simulink model "MenakaModel"  (R2022a)
settings: Solver=ode23tb  StartTime=0.0  StopTime=4  MaxStep=10/(60*24)  RelTol=1e-3
model workspace (MAT data in the model file):
  clima__A_c = 3295.16408265
  clima__A_f = 3100.53942116
  clima__G0 = [0.05; 0.00070738]
  clima__H = 7.9995824611
  clima__T0 = [287.15; 287.15; 287.15; 287.15]
  clima__T_ss = 280.150340169
  clima__alpha_c = 0.0100640347387
  clima__alpha_f = 0.0111385012129
  clima__alpha_i = 0.1
  clima__c_s = [1081 1081]
  clima__cd_c = 8736
  clima__d_c = 1.5
  clima__hour0 = 1
  clima__int_air_speed = 0.5
  clima__l_s = [0.1 0.1]
  clima__lam_s = [2.5 0.85]
  clima__minWindows = 0.299965865643
  clima__rhod_s = [2600 2500]
  clima__tau_c = 1
  crop__A_v = 2080
  crop__C = [0.01 0.001 0.01 0.01]
  crop__C_buf_max = 0.02
  crop__C_wv = 0.2
  crop__Chi_nutrients = [0.015625; 0.0104166666667; 0.00520833333333; 0.00208333333333; 0.00208333333333; 0.00104166666667; 0; 0]
  crop__N = [0; 0; 0; 0; 0; 0; 0; 0]
  crop__R = [0 0 0]
  crop__T_max_v = 40
  crop__T_max_v24 = 27
  crop__T_min_v = 6
  crop__T_min_v24 = 14
  crop__T_sum_end = 1035
  crop__T_v_start_fruit = 1100
  crop__Tsum = 0
  crop__Tv = 288
  crop__b_N_uptake = 0.5
  crop__c_fruit_g = 0.27
  crop__c_fruit_m = 2.3e-07
  crop__c_leaf_g = 0.28
  crop__c_leaf_m = 3.47e-07
  crop__c_stem_g = 0.3
  crop__c_stem_m = 1.47e-07
  crop__fraction_DM = 0.08
  crop__int_air_speed = 0.5
  crop__min_water_capacity = 0.1
  crop__plants_density = 2.1562
  crop__rg_fruit = 2e-07
  crop__rg_leaf = 9.5e-08
  crop__rg_stem = 7.4e-08
  crop__s_buforg_buf = -5000
  crop__s_max_T = 0.5793
  crop__s_max_T24 = 1.3904
  crop__s_min_T = -0.869
  crop__s_min_T24 = -1.1587
  heater__A_e = 0.0001
  heater__A_i = 0.008
  heater__T = 288
  heater__c = 5e-10
  heater__power = 60000000
  screen__Power = 100
  screen__Radthreshold = 900
  screen__beta = 2.23564167038e-14
  screen__gamma_max = 2.26308905438e-14
  screen__velocity = 0.333333333333
  subtrate__C_ws = 0.1
  subtrate__N = [0; 0; 0; 0; 0; 0; 0; 0]
  subtrate__Nmin_subs = 1e-09
  subtrate__Vmax_subs = 10
  subtrate__Vmin_subs = 0.01
  subtrate__sigma_max = 1
  subtrate__sigma_min = 1
  tomato__Cfruit0 = 0.001
  windows__AR = 19.9974923936
  windows__Power = 100
  windows__RadThreshold = 10
  windows__max_night = 10
  windows__tau = 600
undefined symbols (not defined in the file or in its folder): CO2_ppm_ext, Gain_control_Tv_mean, Gain_control_Tv_mean_superior, gain_max_night, GAIN_WIN, Hmax, Hstart, max_night, maxvelocity, RadTh_windows, Radthhold, shift_temp_heat, tau_win, tend_crop1, tend_crop2, tinit_crop1, tinit_crop2, Tmax, Tmax_mean, Tstart, Tven_max, Tven_start, WinAR
libraries: HORTISIM x26, simulink x6
(part 5 of 5)

== matlab function MenakaModel/Control System/PID - constant setpoints - Ti measure/Subsystem1/Triggered Subsystem/MATLAB Function ==
  data: T_min output; T_opt_min output; Tsum input; Rad input; THRad input; T_opt_max output; Tmax output
function [T_min,T_opt_min,T_opt_max,Tmax] = fcn(Tsum, Rad,THRad)


r = OptimalGrowthTemperature(Tsum,Rad,THRad);
r = r + 273.15;

T_min = r(1);
T_opt_min = r(2);
T_opt_max = r(3);
Tmax = r(4);


end
%

function x = OptimalGrowthTemperature(Tsum,Rad,THRad)
    if size(Tsum,2)~=1
       error('Tsum debe ser una columna') 
    end
    x = (Rad> THRad).*OptimalGrowthTemperatureDay(Tsum) + ...
        (Rad<= THRad).*OptimalGrowthTemperatureNight(Tsum);
end


function x = OptimalGrowthTemperatureDay(Tsum)
    if size(Tsum,2)~=1
       error('Tsum debe ser una columna') 
    end
    
%         % Tmin Topt_min Topt_max Tmax
%     x =   [11      18      25     40  ].*theta(400,Tsum) + ...
%           [12      21      24     35  ].*theta(Tsum,400).*theta(1800,Tsum) + ...
%           [15      20      25     30  ].*theta(Tsum,1800);  
%       
              % Tmin Topt_min Topt_max Tmax
    x =   [11      18      35     40  ].*theta(400,Tsum) + ...
          [12      21      30     35  ].*theta(Tsum,400).*theta(1800,Tsum) + ...
          [15      20      30     30  ].*theta(Tsum,1800); 
end

function x = OptimalGrowthTemperatureNight(Tsum)
    if size(Tsum,2)~=1
       error('Tsum debe ser una columna') 
    end
%     x = [11 15 18 30 ].*theta(400,Tsum) + ...
%         [13 14 14 14].*theta(Tsum,400).*theta(1800,Tsum) + ...
%         [10 14 30 35].*theta(Tsum,1800);  
    
        x = [11 15 18 30 ].*theta(400,Tsum) + ...
            [12 13 15 16 ].*theta(Tsum,400).*theta(1800,Tsum) + ...
            [10 14 30 35 ].*theta(Tsum,1800);  
end


function r = theta(x,y)
    eta = 10;
    r = 0.5 + 0.5*tanh(eta*(x-y));
end

== matlab function MenakaModel/Control System/PID - constant setpoints - Ti measure/Subsystem1/Windows Controler/Subsystem/Selection  ==
  data: Rad input; Temperature input; y output; Humidity input; Rad_threshold input
function y = fcn(Rad,Temperature,Humidity,Rad_threshold)

h = double(Rad > Rad_threshold);

y = h*Temperature + (1-h)*Humidity;

%y = Temperature;

== matlab function MenakaModel/Control System/PID-set-points/Subsystem1/Triggered Subsystem/MATLAB Function ==
  data: T_min output; T_opt_min output; Tsum input; Rad input; THRad input; T_opt_max output; Tmax output
function [T_min,T_opt_min,T_opt_max,Tmax] = fcn(Tsum, Rad,THRad)


r = OptimalGrowthTemperature(Tsum,Rad,THRad);
r = r + 273.15;

T_min = r(1);
T_opt_min = r(2);
T_opt_max = r(3);
Tmax = r(4);


end
%

function x = OptimalGrowthTemperature(Tsum,Rad,THRad)
    if size(Tsum,2)~=1
       error('Tsum debe ser una columna') 
    end
    x = (Rad> THRad).*OptimalGrowthTemperatureDay(Tsum) + ...
        (Rad<= THRad).*OptimalGrowthTemperatureNight(Tsum);
end


function x = OptimalGrowthTemperatureDay(Tsum)
    if size(Tsum,2)~=1
       error('Tsum debe ser una columna') 
    end
    
%         % Tmin Topt_min Topt_max Tmax
%     x =   [11      18      25     40  ].*theta(400,Tsum) + ...
%           [12      21      24     35  ].*theta(Tsum,400).*theta(1800,Tsum) + ...
%           [15      20      25     30  ].*theta(Tsum,1800);  
%       
              % Tmin Topt_min Topt_max Tmax
    x =   [11      18      35     40  ].*theta(400,Tsum) + ...
          [12      21      30     35  ].*theta(Tsum,400).*theta(1800,Tsum) + ...
          [15      20      30     30  ].*theta(Tsum,1800); 
end

function x = OptimalGrowthTemperatureNight(Tsum)
    if size(Tsum,2)~=1
       error('Tsum debe ser una columna') 
    end
%     x = [11 15 18 30 ].*theta(400,Tsum) + ...
%         [13 14 14 14].*theta(Tsum,400).*theta(1800,Tsum) + ...
%         [10 14 30 35].*theta(Tsum,1800);  
    
        x = [11 15 18 30 ].*theta(400,Tsum) + ...
            [12 13 15 16 ].*theta(Tsum,400).*theta(1800,Tsum) + ...
            [10 14 30 35 ].*theta(Tsum,1800);  
end


function r = theta(x,y)
    eta = 10;
    r = 0.5 + 0.5*tanh(eta*(x-y));
end

== matlab function MenakaModel/Control System/PID - constant setpoints - Ti measure/Subsystem1/Windows Controler/Subsystem/Ventilation by Hight Humidity ==
  data: HRInt input; y output; HRStart input; HRMax input
function y = fcn(HRInt,HRStart,HRMax)

H1 = HRStart;
H2 = HRMax;
 
y = 100*( 1 - (HRInt-H2)/(H1-H2));

== matlab function MenakaModel/Control System/ON//OFF - constant setpoints/Subsystem1/Windows Controler/Subsystem/Ventilation by Hight Humidity ==
  data: HRInt input; y output; HRStart input; HRMax input
function y = fcn(HRInt,HRStart,HRMax)

H1 = HRStart;
H2 = HRMax;
 
y = 100*( 1 - (HRInt-H2)/(H1-H2));

== matlab function MenakaModel/Control System/ON//OFF - constant setpoints/Subsystem1/Windows Controler/Subsystem/Ventilation by Hight Temperature1 ==
  data: Tstart input; Ti input; y output; Tmax input
function y = fcn(Tstart,Ti,Tmax)

T1 = Tstart;
T2 = Tmax;

y = 100*( 1 - (Ti-T2)/(T1-T2));

== matlab function MenakaModel/Control System/PID - constant setpoints - Ti measure/Subsystem1/Windows Controler/Subsystem/Ventilation by Hight Temperature1 ==
  data: Tstart input; Ti input; y output; Tmax input
function y = fcn(Tstart,Ti,Tmax)

T1 = Tstart;
T2 = Tmax;

y = 100*( 1 - (Ti-T2)/(T1-T2));

== matlab function MenakaModel/Control System/PID - const st - Ti mesure - Dynamics ST/Subsystem1/Triggered Subsystem/MATLAB Function ==
  data: T_min output; T_opt_min output; Tsum input; Rad input; THRad input; T_opt_max output; Tmax output
function [T_min,T_opt_min,T_opt_max,Tmax] = fcn(Tsum, Rad,THRad)


r = OptimalGrowthTemperature(Tsum,Rad,THRad);
r = r + 273.15;

T_min = r(1);
T_opt_min = r(2);
T_opt_max = r(3);
Tmax = r(4);


end
%

function x = OptimalGrowthTemperature(Tsum,Rad,THRad)
    if size(Tsum,2)~=1
       error('Tsum debe ser una columna') 
    end
    x = (Rad> THRad).*OptimalGrowthTemperatureDay(Tsum) + ...
        (Rad<= THRad).*OptimalGrowthTemperatureNight(Tsum);
end


function x = OptimalGrowthTemperatureDay(Tsum)
    if size(Tsum,2)~=1
       error('Tsum debe ser una columna') 
    end
    
%         % Tmin Topt_min Topt_max Tmax
%     x =   [11      18      25     40  ].*theta(400,Tsum) + ...
%           [12      21      24     35  ].*theta(Tsum,400).*theta(1800,Tsum) + ...
%           [15      20      25     30  ].*theta(Tsum,1800);  
%       
              % Tmin Topt_min Topt_max Tmax
    x =   [11      18      35     40  ].*theta(400,Tsum) + ...
          [12      21      30     35  ].*theta(Tsum,400).*theta(1800,Tsum) + ...
          [15      20      30     30  ].*theta(Tsum,1800); 
end

function x = OptimalGrowthTemperatureNight(Tsum)
    if size(Tsum,2)~=1
       error('Tsum debe ser una columna') 
    end
%     x = [11 15 18 30 ].*theta(400,Tsum) + ...
%         [13 14 14 14].*theta(Tsum,400).*theta(1800,Tsum) + ...
%         [10 14 30 35].*theta(Tsum,1800);  
    
        x = [11 15 18 30 ].*theta(400,Tsum) + ...
            [12 13 15 16 ].*theta(Tsum,400).*theta(1800,Tsum) + ...
            [10 14 30 35 ].*theta(Tsum,1800);  
end


function r = theta(x,y)
    eta = 10;
    r = 0.5 + 0.5*tanh(eta*(x-y));
end

== matlab function MenakaModel/Control System/PID - const st - Ti mesure - Dynamics ST/Subsystem1/Windows Controler/Subsystem/Selection  ==
  data: Rad input; Temperature input; y output; Humidity input; Rad_threshold input
function y = fcn(Rad,Temperature,Humidity,Rad_threshold)

h = double(Rad > Rad_threshold);

y = h*Temperature + (1-h)*Humidity;

%y = Temperature;

== matlab function MenakaModel/Control System/PID - const st - Ti mesure - Dynamics ST/Subsystem1/Windows Controler/Subsystem/Ventilation by Hight Humidity ==
  data: HRInt input; y output; HRStart input; HRMax input
function y = fcn(HRInt,HRStart,HRMax)

H1 = HRStart;
H2 = HRMax;
 
y = 100*( 1 - (HRInt-H2)/(H1-H2));

== matlab function MenakaModel/Control System/PID - const st - Ti mesure - Dynamics ST/Subsystem1/Windows Controler/Subsystem/Ventilation by Hight Temperature1 ==
  data: Tstart input; Ti input; y output; Tmax input
function y = fcn(Tstart,Ti,Tmax)

T1 = Tstart;
T2 = Tmax;

y = 100*( 1 - (Ti-T2)/(T1-T2));

== matlab function MenakaModel/Control System/Control System Proportional (Ti) + Tmu /Selector/Windows Controler/Subsystem/Selection  ==
  data: Rad input; Temperature input; y output; Humidity input; Rad_threshold input
function y = fcn(Rad,Temperature,Humidity,Rad_threshold)

h = double(Rad > Rad_threshold);

y = h*Temperature + (1-h)*Humidity;

%y = Temperature;

== matlab function MenakaModel/Control System/Control System Proportional (Ti) + Tmu /Selector/Windows Controler/Subsystem/Ventilation by Hight Humidity ==
  data: HRInt input; y output; HRStart input; HRMax input
function y = fcn(HRInt,HRStart,HRMax)

H1 = HRStart;
H2 = HRMax;
 
y = 100*( 1 - (HRInt-H2)/(H1-H2));

== matlab function MenakaModel/Control System/Control System Proportional (Ti) + Tmu /Selector/Windows Controler/Subsystem/Ventilation by Hight Temperature1 ==
  data: Tstart input; Ti input; y output; Tmax input
function y = fcn(Tstart,Ti,Tmax)

T1 = Tstart;
T2 = Tmax;

y = 100*( 1 - (Ti-T2)/(T1-T2));

== matlab function MenakaModel/Control System/Control System Proportional (Ti) + Tmu Windows Relay/Windows Controler/Subsystem/Selection  ==
  data: Rad input; Temperature input; y output; Humidity input; Rad_threshold input
function y = fcn(Rad,Temperature,Humidity,Rad_threshold)

h = double(Rad > Rad_threshold);

y = h*Temperature + (1-h)*Humidity;

%y = Temperature;

== matlab function MenakaModel/Control System/Setpoints Control - ON//OFF/Subsystem1/Triggered Subsystem/MATLAB Function ==
  data: T_min output; T_opt_min output; Tsum input; Rad input; THRad input; T_opt_max output; Tmax output
function [T_min,T_opt_min,T_opt_max,Tmax] = fcn(Tsum, Rad,THRad)


r = OptimalGrowthTemperature(Tsum,Rad,THRad);
r = r + 273.15;

T_min = r(1);
T_opt_min = r(2);
T_opt_max = r(3);
Tmax = r(4);


end
%

function x = OptimalGrowthTemperature(Tsum,Rad,THRad)
    if size(Tsum,2)~=1
       error('Tsum debe ser una columna') 
    end
    x = (Rad> THRad).*OptimalGrowthTemperatureDay(Tsum) + ...
        (Rad<= THRad).*OptimalGrowthTemperatureNight(Tsum);
end


function x = OptimalGrowthTemperatureDay(Tsum)
    if size(Tsum,2)~=1
       error('Tsum debe ser una columna') 
    end
    
%         % Tmin Topt_min Topt_max Tmax
%     x =   [11      18      25     40  ].*theta(400,Tsum) + ...
%           [12      21      24     35  ].*theta(Tsum,400).*theta(1800,Tsum) + ...
%           [15      20      25     30  ].*theta(Tsum,1800);  
%       
              % Tmin Topt_min Topt_max Tmax
    x =   [11      18      35     40  ].*theta(400,Tsum) + ...
          [12      21      30     35  ].*theta(Tsum,400).*theta(1800,Tsum) + ...
          [15      20      30     30  ].*theta(Tsum,1800); 
end

function x = OptimalGrowthTemperatureNight(Tsum)
    if size(Tsum,2)~=1
       error('Tsum debe ser una columna') 
    end
%     x = [11 15 18 30 ].*theta(400,Tsum) + ...
%         [13 14 14 14].*theta(Tsum,400).*theta(1800,Tsum) + ...
%         [10 14 30 35].*theta(Tsum,1800);  
    
        x = [11 15 18 30 ].*theta(400,Tsum) + ...
            [12 13 15 16 ].*theta(Tsum,400).*theta(1800,Tsum) + ...
            [10 14 30 35 ].*theta(Tsum,1800);  
end


function r = theta(x,y)
    eta = 10;
    r = 0.5 + 0.5*tanh(eta*(x-y));
end

== matlab function MenakaModel/Control System/Control System Proportional (Ti) + Tmu Windows Relay/Windows Controler/Subsystem/Ventilation by Hight Humidity ==
  data: HRInt input; y output; HRStart input; HRMax input
function y = fcn(HRInt,HRStart,HRMax)

H1 = HRStart;
H2 = HRMax;
 
y = 100*( 1 - (HRInt-H2)/(H1-H2));

== matlab function MenakaModel/Control System/Setpoints Control - ON//OFF/Subsystem1/Windows Controler/Subsystem/Selection  ==
  data: Rad input; Temperature input; y output; Humidity input; Rad_threshold input
function y = fcn(Rad,Temperature,Humidity,Rad_threshold)

h = double(Rad > Rad_threshold);

y = h*Temperature + (1-h)*Humidity;

%y = Temperature;

== matlab function MenakaModel/Control System/Setpoints Control - ON//OFF/Subsystem1/Windows Controler/Subsystem/Ventilation by Hight Humidity ==
  data: HRInt input; y output; HRStart input; HRMax input
function y = fcn(HRInt,HRStart,HRMax)

H1 = HRStart;
H2 = HRMax;
 
y = 100*( 1 - (HRInt-H2)/(H1-H2));

== matlab function MenakaModel/Control System/Setpoints Control - ON//OFF/Subsystem1/Windows Controler/Subsystem/Ventilation by Hight Temperature1 ==
  data: Tstart input; Ti input; y output; Tmax input
function y = fcn(Tstart,Ti,Tmax)

T1 = Tstart;
T2 = Tmax;

y = 100*( 1 - (Ti-T2)/(T1-T2));

== matlab function MenakaModel/Control System/PID-set-points/Subsystem1/Windows Controler/Subsystem/Selection  ==
  data: Rad input; Temperature input; y output; Humidity input; Rad_threshold input
function y = fcn(Rad,Temperature,Humidity,Rad_threshold)

h = double(Rad > Rad_threshold);

y = h*Temperature + (1-h)*Humidity;

%y = Temperature;

== matlab function MenakaModel/Control System/PID-set-points/Subsystem1/Windows Controler/Subsystem/Ventilation by Hight Humidity ==
  data: HRInt input; y output; HRStart input; HRMax input
function y = fcn(HRInt,HRStart,HRMax)

H1 = HRStart;
H2 = HRMax;
 
y = 100*( 1 - (HRInt-H2)/(H1-H2));

== matlab function MenakaModel/Control System/PID-set-points/Subsystem1/Windows Controler/Subsystem/Ventilation by Hight Temperature1 ==
  data: Tstart input; Ti input; y output; Tmax input
function y = fcn(Tstart,Ti,Tmax)

T1 = Tstart;
T2 = Tmax;

y = 100*( 1 - (Ti-T2)/(T1-T2));

== matlab function MenakaModel/Control System/PID - constant setpoints/Subsystem1/Triggered Subsystem/MATLAB Function ==
  data: T_min output; T_opt_min output; Tsum input; Rad input; THRad input; T_opt_max output; Tmax output
function [T_min,T_opt_min,T_opt_max,Tmax] = fcn(Tsum, Rad,THRad)


r = OptimalGrowthTemperature(Tsum,Rad,THRad);
r = r + 273.15;

T_min = r(1);
T_opt_min = r(2);
T_opt_max = r(3);
Tmax = r(4);


end
%

function x = OptimalGrowthTemperature(Tsum,Rad,THRad)
    if size(Tsum,2)~=1
       error('Tsum debe ser una columna') 
    end
    x = (Rad> THRad).*OptimalGrowthTemperatureDay(Tsum) + ...
        (Rad<= THRad).*OptimalGrowthTemperatureNight(Tsum);
end


function x = OptimalGrowthTemperatureDay(Tsum)
    if size(Tsum,2)~=1
       error('Tsum debe ser una columna') 
    end
    
%         % Tmin Topt_min Topt_max Tmax
%     x =   [11      18      25     40  ].*theta(400,Tsum) + ...
%           [12      21      24     35  ].*theta(Tsum,400).*theta(1800,Tsum) + ...
%           [15      20      25     30  ].*theta(Tsum,1800);  
%       
              % Tmin Topt_min Topt_max Tmax
    x =   [11      18      35     40  ].*theta(400,Tsum) + ...
          [12      21      30     35  ].*theta(Tsum,400).*theta(1800,Tsum) + ...
          [15      20      30     30  ].*theta(Tsum,1800); 
end

function x = OptimalGrowthTemperatureNight(Tsum)
    if size(Tsum,2)~=1
       error('Tsum debe ser una columna') 
    end
%     x = [11 15 18 30 ].*theta(400,Tsum) + ...
%         [13 14 14 14].*theta(Tsum,400).*theta(1800,Tsum) + ...
%         [10 14 30 35].*theta(Tsum,1800);  
    
        x = [11 15 18 30 ].*theta(400,Tsum) + ...
            [12 13 15 16 ].*theta(Tsum,400).*theta(1800,Tsum) + ...
            [10 14 30 35 ].*theta(Tsum,1800);  
end


function r = theta(x,y)
    eta = 10;
    r = 0.5 + 0.5*tanh(eta*(x-y));
end

== matlab function MenakaModel/Control System/PID - constant setpoints/Subsystem1/Windows Controler/Subsystem/Selection  ==
  data: Rad input; Temperature input; y output; Humidity input; Rad_threshold input
function y = fcn(Rad,Temperature,Humidity,Rad_threshold)

h = double(Rad > Rad_threshold);

y = h*Temperature + (1-h)*Humidity;

%y = Temperature;

== matlab function MenakaModel/Control System/PID - constant setpoints/Subsystem1/Windows Controler/Subsystem/Ventilation by Hight Humidity ==
  data: HRInt input; y output; HRStart input; HRMax input
function y = fcn(HRInt,HRStart,HRMax)

H1 = HRStart;
H2 = HRMax;
 
y = 100*( 1 - (HRInt-H2)/(H1-H2));

== matlab function MenakaModel/Control System/PID - constant setpoints/Subsystem1/Windows Controler/Subsystem/Ventilation by Hight Temperature1 ==
  data: Tstart input; Ti input; y output; Tmax input
function y = fcn(Tstart,Ti,Tmax)

T1 = Tstart;
T2 = Tmax;

y = 100*( 1 - (Ti-T2)/(T1-T2));
